simulink model "FLIGHT_hexacopter"  (R2024a)
settings: Solver=FixedStepDiscrete  StartTime=0.0  StopTime=inf  FixedStep=SampleTime_SAS  RelTol=1e-3  EnableMultiTasking=on
InitFcn:
  | Init_FLIGHT_Hexacopter
values from neighbouring files (symbols this model uses):
  d2r = pi/180    (= 0.0174532925199)    [Init_FLIGHT_Hexacopter.m]
  Kdpr = 0.004    [Init_FLIGHT_Hexacopter_fromNCMS.m]
  Kdrr = 0.004    [Init_FLIGHT_Hexacopter_fromNCMS.m]
  Kdvz = 0.0254    [Init_FLIGHT_Hexacopter_fromNCMS.m]
  Kdyr = 0.0298    [Init_FLIGHT_Hexacopter_fromNCMS.m]
  Kipr = 0.0    (= 0)    [Init_FLIGHT_Hexacopter_fromNCMS.m]
  Kirr = 0.0    (= 0)    [Init_FLIGHT_Hexacopter_fromNCMS.m]
  Kivz = 0.6304    [Init_FLIGHT_Hexacopter_fromNCMS.m]
  Kiyr = 0.0    (= 0)    [Init_FLIGHT_Hexacopter_fromNCMS.m]
  Kpp = 3.3894    [Init_FLIGHT_Hexacopter_fromNCMS.m]
  Kppr = 0.1    [Init_FLIGHT_Hexacopter_fromNCMS.m]
  Kpr = 3.3894    [Init_FLIGHT_Hexacopter_fromNCMS.m]
  Kprr = 0.1    [Init_FLIGHT_Hexacopter_fromNCMS.m]
  Kpvz = 0.3191    [Init_FLIGHT_Hexacopter_fromNCMS.m]
  Kpyr = 0.3744    [Init_FLIGHT_Hexacopter_fromNCMS.m]
  MAX_CONTROL_ANGLE_PITCH = 30*pi/180    (= 0.523598775598)    [Init_FLIGHT_Hexacopter.m]    (also in Init_FLIGHT_Hexacopter_fromNCMS.m = 0.349065850399)
  MAX_CONTROL_ANGLE_RATE_PITCH = 360*pi/180    (= 6.28318530718)    [Init_FLIGHT_Hexacopter.m]    (also in Init_FLIGHT_Hexacopter_fromNCMS.m)
  MAX_CONTROL_ANGLE_RATE_ROLL = 360*pi/180    (= 6.28318530718)    [Init_FLIGHT_Hexacopter.m]    (also in Init_FLIGHT_Hexacopter_fromNCMS.m)
  MAX_CONTROL_ANGLE_RATE_Y = 120*pi/180    (= 2.09439510239)    [Init_FLIGHT_Hexacopter.m]    (also in Init_FLIGHT_Hexacopter_fromNCMS.m)
  MAX_CONTROL_ANGLE_ROLL = 30*pi/180    (= 0.523598775598)    [Init_FLIGHT_Hexacopter.m]    (also in Init_FLIGHT_Hexacopter_fromNCMS.m = 0.349065850399)
  MAX_CONTROL_VELOCITY_XY = 1.5    [Init_FLIGHT_Hexacopter.m]    (also in Init_FLIGHT_Hexacopter_fromNCMS.m)
  MAX_CONTROL_VELOCITY_Z = 1    [Init_FLIGHT_Hexacopter.m]    (also in Init_FLIGHT_Hexacopter_fromNCMS.m)
  Npr = 50    [Init_FLIGHT_Hexacopter_fromNCMS.m]
  Nrr = 50    [Init_FLIGHT_Hexacopter_fromNCMS.m]
  Nvz = Npr    (= 50)    [Init_FLIGHT_Hexacopter_fromNCMS.m]
  Nyr = 50    [Init_FLIGHT_Hexacopter_fromNCMS.m]
  SampleTime = 1/200    (= 0.005)    [Init_FLIGHT_Hexacopter.m]    (also in Init_FLIGHT_Hexacopter_fromNCMS.m = 0.01)
  SampleTime_SAS = 1/1000    (= 0.001)    [Init_FLIGHT_Hexacopter.m]
undefined symbols (not defined in the file or in its folder): arguments, event_sequence, id, log_levels, MPC_Z_D, MPC_Z_I, MPC_Z_P, noutputs, output, pitch, pitch_body, q_d, roll, roll_body, thrust_body, timestamp, vx, vy, vz, x, y, yaw, yaw_sp_move_rate, z
libraries: px4lib x35, px4uORBlib x12, px4Utilslib x11, slpidlib x10, simulink x3, simulink_extras x2, px4Sensorslib x2, sharedtransform x1
(part 1 of 3)
settings Model: SimulationMode=external  ExtModeTrigDuration=10  Creator=user  LastModifiedBy=sslee
settings SolverCC: AlgebraicLoopSolver=TrustRegion  PositivePriorityOrder=on  MaxZcPerStep=1
settings OptimizationCC: DefaultUnderspecifiedDataType=single  EnhancedBackFolding=on  PassReuseOutputArgsAs=Individual arguments  ZeroExternalMemoryAtStartup=off  ZeroInternalMemoryAtStartup=off  MaxStackSize=64  OptimizeBlockOrder=speed  DifferentSizesBufferReuse=on  OptimizationCustomize=off  EfficientTunableParamExpr=on
settings DebuggingCC: ParameterTunabilityLossMsg=error  UnconnectedInputMsg=warning  UnconnectedOutputMsg=warning  UnconnectedLineMsg=warning
settings HardwareCC: ProdBitPerPointer=32  ProdBitPerSizeT=32  ProdBitPerPtrDiffT=32  ProdLargestAtomicInteger=Long  ProdLargestAtomicFloat=Double  ProdWordSize=32  ProdLongLongMode=on  ProdHWDeviceType=ARM Compatible->ARM Cortex
settings ModelReferenceCC: EnableRefExpFcnMdlSchedulingChecks=on
settings SFSimCC: MATLABDynamicMemAlloc=off  SimTargetLang=C++
settings RTWCC: Description=Embedded Coder  SystemTargetFile=ert.tlc  HardwareBoard=PX4 Pixhawk 6x  TLCOptions="-aInlineSetEventsForThisBaseRateFcn=TLC_FALSE -aSuppressMultiTaskScheduler=TLC_FALSE  -aRateBasedStepFcn=0"  TemplateMakefile=ert_default_tmf  GenerateReport=on  Toolchain=GNU Tools for PX4 Autopilots  TargetLang=C++  GPUComputeCapability=3.5  DLArmComputeVersion=19.05
settings CodeAppCC: ForceParamTrailComments=on  IgnoreCustomStorageClasses=off  OperatorAnnotations=on  SimulinkDataObjDesc=on  SFDataObjDesc=on  MATLABFcnDesc=on  InsertBlockDesc=on
settings ERTTargetCC: SupportVariableSizeSignals=on  ExtModeTransport=3  ExtModeStaticAlloc=on  ExtModeStaticAllocSize=1024  ExtModeMexFile=ext_xcp  ExtModeIntrfLevel=Level2 - Open

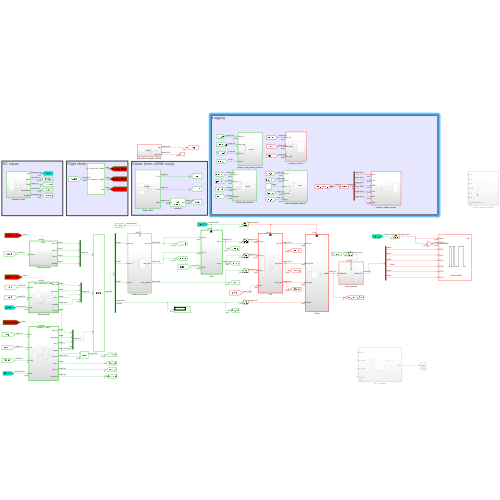
[thumbnail: Simulink's stored preview of the top-level diagram]
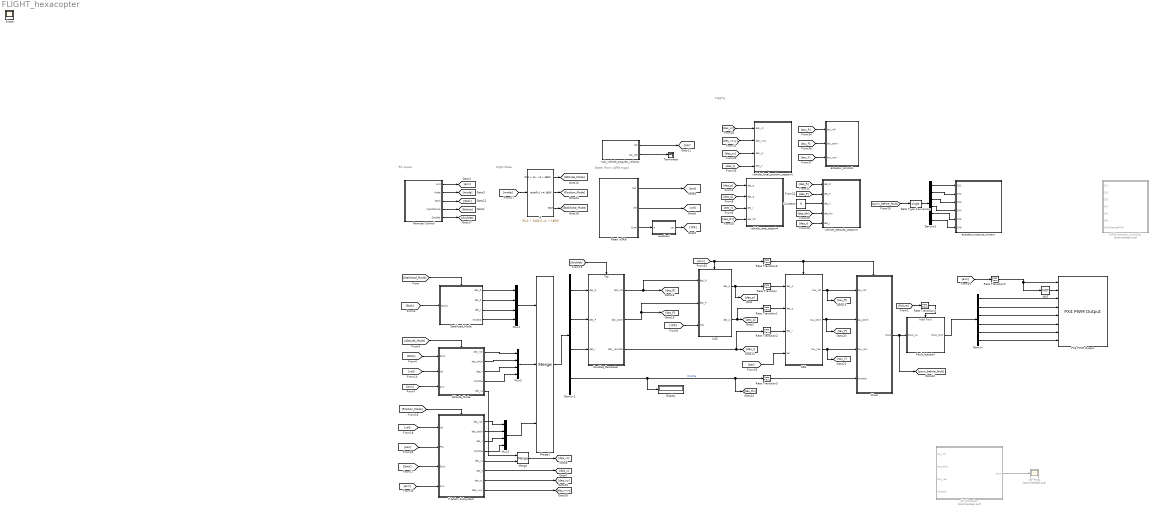
== system FLIGHT_hexacopter ==
  note: States (from uORB msgs)
  note: Logging
  note: Flight Mode
  note: RC inputs
  Altitude_Mode : Subsystem
  CAS : Subsystem
  Constant : Constant  Value=0  OutDataTypeStr=single  SampleTime=SampleTime
  Data Type Conversion : DataTypeConversion  OutDataTypeStr=single  SaturateOnIntegerOverflow=off  RndMeth=Floor
  Demux : Demux  Outputs=6
  Demux1 : Demux
  Demux3 : Demux  Outputs=6
  Display : Display
  Doublet_Generator : Subsystem
      settings: PortSchema="{\"entries\":[{\"content\":{\"sides\":[{\"content\":{\"connectorIds\":[\"In1\",\"In2\",\"In3\"]},\"type\":\"ConnectorPlacement.EquallySpacedRectSide\",\"uuid\":\"ec38b5d1-b3a9-4497-90eb-b31f6af6263d\"},{\"content\":{\"connectorIds\":[\"Out1\",\"Out2\",\"Out3\"],\"side\":\"RIGHT\"},\"type\":\"ConnectorPlacement.EquallySpacedRectSide\",\"uuid\":\"b680dd4c-5362-4b07-9f32-4954453bae35\"},{\"content\":{\"connectorIds\":[\"In4\"],\"side\":\"TOP\"},\"type\":\"ConnectorPlacement.EquallySpacedRectSide\",\"uuid\":\"c853e1a7-4b20-4202-99cf-4bec5916d7ea\"}]},\"type\":\"ConnectorPlacement.EquallySpacedConnector\",\"uuid\":\"c3796ba1-a87a-49a7-b842-2bb0a159edd5\"}],\"packageUris\":[\"http://schema.mathworks.com/mf0/Connector/R2020b\"],\"version\":\"1.0\"}"
  Fault_Injection : Subsystem
      settings: PortSchema="{\"entries\":[{\"content\":{\"sides\":[{\"content\":{\"connectorIds\":[\"In1\"]},\"type\":\"ConnectorPlacement.EquallySpacedRectSide\",\"uuid\":\"fab26c65-8d77-46b7-b375-2033d08e8306\"},{\"content\":{\"connectorIds\":[\"Out1\"],\"side\":\"RIGHT\"},\"type\":\"ConnectorPlacement.EquallySpacedRectSide\",\"uuid\":\"bc3f50bd-e170-4b75-8089-4f92da68e83e\"},{\"content\":{\"connectorIds\":[\"In2\"],\"side\":\"TOP\"},\"type\":\"ConnectorPlacement.EquallySpacedRectSide\",\"uuid\":\"873ada90-6f93-48ab-a701-a52d28357753\"}]},\"type\":\"ConnectorPlacement.EquallySpacedConnector\",\"uuid\":\"201be8b3-bff4-4924-8e0c-28e5fee33d1c\"}],\"packageUris\":[\"http://schema.mathworks.com/mf0/Connector/R2020b\"],\"version\":\"1.0\"}"
  If : If  IfExpression=u1 > 1400 & u1 < 1800  ElseIfExpressions=u1 >= 1800
  If Action Subsystem : Subsystem  TreatAsAtomicUnit=on
  Merge : Merge
  Merge1 : Merge  Inputs=3
  Mixer : Subsystem
  Mux1 : Mux
  Mux2 : Mux
  Mux3 : Mux
  NOT : Logic  Operator=NOT  IconShape=distinctive  AllPortsSameDT=off  OutDataTypeStr=boolean
  PX4 PWM Output : px4lib/PX4 PWM Output  pwmDevice=Main  pwmChannel1_=on  pwmChannel2_=on  pwmChannel3_=on  pwmChannel4_=on  pwmChannel5_=on  pwmChannel6_=on  pwmChannel7_=off  pwmChannel8_=off
      settings: SourceProductName=UAV Toolbox Support Package for PX4 Autopilots
  QP PWM : Scope  Commented=on
  QP_Allocation : Subsystem  Commented=on
  Rate Transition{,1..6} (7 alike) : RateTransition  OutPortSampleTime=SampleTime_SAS
  Read uORB : Subsystem
  Remote Control : Subsystem
  SAS : Subsystem
  Stabilized_Mode : Subsystem  TreatAsAtomicUnit=on
  Terminator : Terminator
  actuator_controls : Subsystem
  actuator_outputs_motors : Subsystem
  quat2eul : MATLAB Function  TreatAsAtomicUnit=on
  sub_vehicle_angular_velocity : Subsystem
  uORB_actuator_outputs1 : Subsystem  Commented=on
  vehicle_attitude_setpoint : Subsystem
  vehicle_local_position_setpoint : Subsystem
  vehicle_rate_setpoint : Subsystem
  Scope : Scope
  wires:
  Remote Control/4(InjectFailure) -> [failure]
  Stabilized_Mode/4(throttle) -> Mux1/4
  quat2eul/1(ypr) -> [YPR]
  [YPR] -> CAS/3(YPR)
  [mode] -> If/1
  sub_vehicle_angular_velocity/1(pqr) -> [pqr]
  [pqr] -> SAS/4(pqr)
  Read uORB/2(Vel) -> [vel]
  Mux1/1 -> Merge1/1
  Stabilized_Mode/2(des_P) -> Mux1/2
  Altitude_Mode/1(des_roll) -> Mux2/1
  Stabilized_Mode/1(des_R) -> Mux1/1
  Remote Control/2(Mode) -> [mode]
  Read uORB/3(Quat) -> quat2eul/1(q)
  Stabilized_Mode/3(des_r) -> Mux1/3
  Mux2/1 -> Merge1/2
  Altitude_Mode/3(des_r) -> Mux2/3
  Altitude_Mode/2(des_pitch) -> Mux2/2
  Demux1/4 -> Display/1, Rate Transition3/1, [des_thr]  "throttle"
  [Stick] -> Stabilized_Mode/1(Sticks)
  SAS/2(tau_pitch) -> [tau_P], Mixer/2(tau_pitch)
  SAS/1(tau_roll) -> [tau_R], Mixer/1(tau_roll)
  Remote Control/1(Arm) -> [arm]
  [Stick] -> Altitude_Mode/1(Stick)
  [Stabilized_Mode] -> Stabilized_Mode/Action
  [vel] -> Altitude_Mode/2(vel)
  SAS/3(tau_yaw) -> [tau_Y], Mixer/3(tau_yaw)
  If/1 -> [Altitude_Mode]
  CAS/1(des_p) -> [des_p], Rate Transition/1
  Merge1/1 -> Demux1/1
  If/3 -> [Stabilized_Mode]
  CAS/2(des_q) -> [des_q], Rate Transition1/1
  Fault_Injection/1(PWM_OUT) -> Demux/1
  Read uORB/1(Pos) -> [pos]
  Remote Control/3(Stick) -> [Stick]
  [Altitude_Mode] -> Altitude_Mode/Action
  [des_p] -> vehicle_rate_setpoint/1(des_p)
  [des_q] -> vehicle_rate_setpoint/2(des_q)
  [des_r] -> vehicle_rate_setpoint/3(des_r)
  [des_thr] -> vehicle_rate_setpoint/4(des_thr)
  Altitude_Mode/4(throttle) -> Mux2/4
  QP_Allocation/1(pwm) -> QP PWM/1
  Mixer/1(PWM) -> [pwm_before_fault], Fault_Injection/1(PWM_IN)
  Remote Control/5(Doublet) -> [doublet]
  [des_P] -> vehicle_attitude_setpoint/2(des_P)
  [des_R] -> vehicle_attitude_setpoint/1(des_R)
  [des_thr] -> vehicle_attitude_setpoint/4(des_thr)
  [des_r] -> vehicle_attitude_setpoint/5(des_r)
  [arm] -> Rate Transition5/1
  Demux/1 -> PX4 PWM Output/3
  Demux/2 -> PX4 PWM Output/4
  Demux/3 -> PX4 PWM Output/5
  Demux/4 -> PX4 PWM Output/6
  Demux/5 -> PX4 PWM Output/7
  Demux/6 -> PX4 PWM Output/8
  NOT/1 -> PX4 PWM Output/2
  Constant/1 -> vehicle_attitude_setpoint/3(des_Y)
  [pwm_before_fault] -> Data Type Conversion/1
  If/2 -> [Position_Mode]
  [Position_Mode] -> If Action Subsystem/Action
  [vel] -> If Action Subsystem/1(vel)
  If Action Subsystem/1(des_roll) -> Mux3/1
  If Action Subsystem/2(des_pitch) -> Mux3/2
  If Action Subsystem/3(des_r) -> Mux3/3
  If Action Subsystem/4(throttle) -> Mux3/4
  Mux3/1 -> Merge1/3
  Merge/1 -> [des_vz]
  Altitude_Mode/5(des_vz) -> Merge/1
  [des_vz] -> vehicle_local_position_setpoint/1(des_vz)
  [Stick] -> If Action Subsystem/3(Stick)
  [pos] -> If Action Subsystem/2(Pos)
  If Action Subsystem/5(des_vz) -> Merge/2
  If Action Subsystem/6(des_z) -> [des_z]
  If Action Subsystem/7(des_xy) -> [des_xy]
  If Action Subsystem/8(des_vxvy) -> [des_vxvy]
  [des_vxvy] -> vehicle_local_position_setpoint/2(des_vxvy)
  [des_xy] -> vehicle_local_position_setpoint/3(des_xy)
  [des_z] -> vehicle_local_position_setpoint/4(des_z)
  Data Type Conversion/1 -> Demux3/1
  [arm] -> Rate Transition6/1, CAS/Enable
  [arm] -> If Action Subsystem/4(arm)
  [arm] -> Altitude_Mode/3(arm)
  Demux3/1 -> actuator_outputs_motors/1(Ch1)
  Demux3/2 -> actuator_outputs_motors/2(Ch2)
  Demux3/3 -> actuator_outputs_motors/3(Ch3)
  Demux3/4 -> actuator_outputs_motors/4(Ch4)
  Demux3/5 -> actuator_outputs_motors/5(Ch5)
  Demux3/6 -> actuator_outputs_motors/6(Ch6)
  [tau_R] -> actuator_controls/1(tau_roll)
  [tau_P] -> actuator_controls/2(tau_pitch)
  [tau_Y] -> actuator_controls/3(tau_yaw)
  Demux1/1 -> Doublet_Generator/1(des_R)
  Demux1/2 -> Doublet_Generator/2(des_P)
  Demux1/3 -> Doublet_Generator/3(des_r)
  Doublet_Generator/1(des_roll) -> CAS/1(des_R), [des_R]
  Doublet_Generator/2(des_pitch) -> [des_P], CAS/2(des_P)
  Doublet_Generator/3(des_yawrate) -> [des_r], Rate Transition2/1
  [doublet] -> Doublet_Generator/4(flag)
  Rate Transition/1 -> SAS/1(des_p)
  Rate Transition1/1 -> SAS/2(des_q)
  Rate Transition2/1 -> SAS/3(des_r)
  Rate Transition3/1 -> Mixer/4(throttle)
  [failure] -> Rate Transition4/1
  Rate Transition4/1 -> Fault_Injection/2(Inject Fault)
  Rate Transition5/1 -> NOT/1, PX4 PWM Output/1
  Rate Transition6/1 -> SAS/Enable, Mixer/Enable
  sub_vehicle_angular_velocity/2(pqr_dot) -> Terminator/1

== system FLIGHT_hexacopter/Altitude_Mode ==
  Stick : Inport
  vel : Inport  Port=2
  arm : Inport  Port=3
  Action Port : ActionPort  ActionPortLabel=if(u1 > 1400 & u1 < 1800)
  Altitude_Mode_Stick2Command : Subsystem
  Demux2 : Demux  Outputs=3
  Terminator2 : Terminator
  Terminator3 : Terminator
  Vz Controller : Subsystem
  des_roll : Outport
  des_pitch : Outport  Port=2
  des_r : Outport  Port=3
  throttle : Outport  Port=4
  des_vz : Outport  Port=5
  wires:
  Stick/1 -> Altitude_Mode_Stick2Command/1(Stick)
  Vz Controller/1(throttle) -> throttle/1
  Demux2/3 -> Vz Controller/2(vz)
  vel/1 -> Demux2/1
  Altitude_Mode_Stick2Command/3(des_r) -> des_r/1
  Demux2/1 -> Terminator2/1
  Demux2/2 -> Terminator3/1
  Altitude_Mode_Stick2Command/2(des_pitch) -> des_pitch/1
  Altitude_Mode_Stick2Command/4(des_vz) -> des_vz/1, Vz Controller/1(des_vz)
  arm/1 -> Vz Controller/Enable
  Altitude_Mode_Stick2Command/1(des_roll) -> des_roll/1

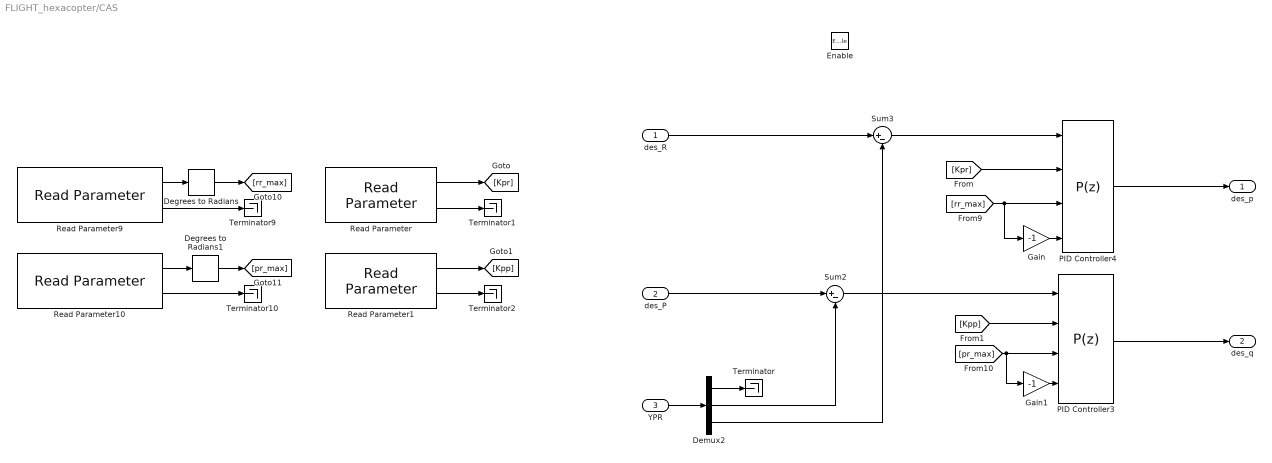
== system FLIGHT_hexacopter/CAS ==
  des_R : Inport
  des_P : Inport  Port=2
  YPR : Inport  Port=3
  Enable : EnablePort
  Degrees to Radians : simulink_extras/Transformations/Degrees to Radians
  Degrees to Radians1 : simulink_extras/Transformations/Degrees to Radians
  Demux2 : Demux  Outputs=3
  Gain : Gain  Gain=-1
  Gain1 : Gain  Gain=-1
  PID Controller3 : slpidlib/PID Controller  Controller=P  Form=Parallel  TimeDomain=Discrete-time  UseExternalTs=off  SampleTime=SampleTime  IntegratorMethod=Forward Euler  FilterMethod=Forward Euler  ControllerParametersSource=external  P=Kpp  I=1  UseKiTs=off  D=0  UseExternalDerivativeSource=off  N=100  UseFilter=on  TunerSelectOption=Transfer Function Based (PID Tuner App)  InitialConditionSource=internal  InitialConditionForIntegrator=0  InitialConditionForFilter=0  DifferentiatorICPrevScaledInput=0  ExternalReset=none  TrackingMode=off  Kt=1  LimitOutput=on  SatLimitsSource=external  UpperSaturationLimit=MAX_CONTROL_ANGLE_RATE_PITCH  LowerSaturationLimit=-MAX_CONTROL_ANGLE_RATE_PITCH  LinearizeAsGain=on  AntiWindupMode=none  Kb=1  LimitIntegrator=off  UpperIntegratorSaturationLimit=inf  LowerIntegratorSaturationLimit=-inf  POutMin=[]  POutMax=[]  IOutMin=[]  IOutMax=[]  DOutMin=[]  DOutMax=[]  NOutMin=[]  NOutMax=[]  SumOutMin=[]  SumOutMax=[]  SaturationOutMin=[]  SaturationOutMax=[]  PParamMin=[]  PParamMax=[]  IParamMin=[]  IParamMax=[]  DParamMin=[]  DParamMax=[]  NParamMin=[]  NParamMax=[]  KbParamMin=[]  KbParamMax=[]  KtParamMin=[]  KtParamMax=[]  KbOutMin=[]  KbOutMax=[]  KtOutMin=[]  KtOutMax=[]  IntegratorOutMin=[]  IntegratorOutMax=[]  FilterOutMin=[]  FilterOutMax=[]  SumI1OutMin=[]  SumI1OutMax=[]  SumI2OutMin=[]  SumI2OutMax=[]  SumI3OutMin=[]  SumI3OutMax=[]  SumI4OutMin=[]  SumI4OutMax=[]  SumDOutMin=[]  SumDOutMax=[]  DifferentiatorOutMin=[]  DifferentiatorOutMax=[]  FilterDiffOutCoefMin=[]  FilterDiffOutCoefMax=[]  ReciprocalOutMin=[]  ReciprocalOutMax=[]  SumDenOutMin=[]  SumDenOutMax=[]  SumNumOutMin=[]  SumNumOutMax=[]  DivideOutMin=[]  DivideOutMax=[]  UdiffTsProdOutMin=[]  UdiffTsProdOutMax=[]  NTsProdOutMin=[]  NTsProdOutMax=[]  UintegralTsProdOutMin=[]  UintegralTsProdOutMax=[]  UngainTsProdOutMin=[]  UngainTsProdOutMax=[]  ClampingZeroOutDataTypeStr=Inherit: Inherit via back propagation  ClampingZeroOutMin=[]  ClampingZeroOutMax=[]  FilterDenConstantOutDataTypeStr=Inherit: Inherit via back propagation  FilterDenConstantOutMin=[]  FilterDenConstantOutMax=[]  PCopyOutDataTypeStr=Inherit: Inherit via back propagation  PCopyOutMin=[]  PCopyOutMax=[]  NCopyOutDataTypeStr=Inherit: Inherit via back propagation  NCopyOutMin=[]  NCopyOutMax=[]  IntegratorContinuousStateAttributes=''  IntegratorStateMustResolveToSignalObject=off  IntegratorRTWStateStorageClass=Auto  FilterContinuousStateAttributes=''  FilterStateMustResolveToSignalObject=off  FilterRTWStateStorageClass=Auto  ParallelPVariant=ExternalParameters  IdealPVariant=Disabled  IVariant=Disabled  DVariant=Disabled  IntegratorVariant=Disabled  SatVariant=External  AWVariant=Disabled  PCopyVariant=Disabled  TRVariant=Disabled  FdbkBlocksVariant=Forward  IdealPFdbkVariant=Disabled  SatFdbkVariant=Disabled  DerivativeFilterVariant=Disabled  NVariant=Disabled  NCopyVariant=Disabled_SignalSpec  FilterICVariant=Disabled  IntegratorICVariant=Disabled  ExternalResetVariant=Disabled  TRSumVariant=Passthrough  SumFdbkVariant=Disabled  SumVariant=Passthrough_P  TsampFilterVariant=InternalTs  TsampNgainVariant=Passthrough  TsampIntegralVariant=Disabled_SignalSpec  ExternalSaturationOutDataTypeStr=Inherit: Same as second input  DerivativeSourceVariant=Disabled
  PID Controller4 : slpidlib/PID Controller  Controller=P  Form=Parallel  TimeDomain=Discrete-time  UseExternalTs=off  SampleTime=SampleTime  IntegratorMethod=Forward Euler  FilterMethod=Forward Euler  ControllerParametersSource=external  P=Kpr  I=1  UseKiTs=off  D=0  UseExternalDerivativeSource=off  N=100  UseFilter=on  TunerSelectOption=Transfer Function Based (PID Tuner App)  InitialConditionSource=internal  InitialConditionForIntegrator=0  InitialConditionForFilter=0  DifferentiatorICPrevScaledInput=0  ExternalReset=none  TrackingMode=off  Kt=1  LimitOutput=on  SatLimitsSource=external  UpperSaturationLimit=MAX_CONTROL_ANGLE_RATE_ROLL  LowerSaturationLimit=-MAX_CONTROL_ANGLE_RATE_ROLL  LinearizeAsGain=on  AntiWindupMode=none  Kb=1  LimitIntegrator=off  UpperIntegratorSaturationLimit=inf  LowerIntegratorSaturationLimit=-inf  POutMin=[]  POutMax=[]  IOutMin=[]  IOutMax=[]  DOutMin=[]  DOutMax=[]  NOutMin=[]  NOutMax=[]  SumOutMin=[]  SumOutMax=[]  SaturationOutMin=[]  SaturationOutMax=[]  PParamMin=[]  PParamMax=[]  IParamMin=[]  IParamMax=[]  DParamMin=[]  DParamMax=[]  NParamMin=[]  NParamMax=[]  KbParamMin=[]  KbParamMax=[]  KtParamMin=[]  KtParamMax=[]  KbOutMin=[]  KbOutMax=[]  KtOutMin=[]  KtOutMax=[]  IntegratorOutMin=[]  IntegratorOutMax=[]  FilterOutMin=[]  FilterOutMax=[]  SumI1OutMin=[]  SumI1OutMax=[]  SumI2OutMin=[]  SumI2OutMax=[]  SumI3OutMin=[]  SumI3OutMax=[]  SumI4OutMin=[]  SumI4OutMax=[]  SumDOutMin=[]  SumDOutMax=[]  DifferentiatorOutMin=[]  DifferentiatorOutMax=[]  FilterDiffOutCoefMin=[]  FilterDiffOutCoefMax=[]  ReciprocalOutMin=[]  ReciprocalOutMax=[]  SumDenOutMin=[]  SumDenOutMax=[]  SumNumOutMin=[]  SumNumOutMax=[]  DivideOutMin=[]  DivideOutMax=[]  UdiffTsProdOutMin=[]  UdiffTsProdOutMax=[]  NTsProdOutMin=[]  NTsProdOutMax=[]  UintegralTsProdOutMin=[]  UintegralTsProdOutMax=[]  UngainTsProdOutMin=[]  UngainTsProdOutMax=[]  ClampingZeroOutDataTypeStr=Inherit: Inherit via back propagation  ClampingZeroOutMin=[]  ClampingZeroOutMax=[]  FilterDenConstantOutDataTypeStr=Inherit: Inherit via back propagation  FilterDenConstantOutMin=[]  FilterDenConstantOutMax=[]  PCopyOutDataTypeStr=Inherit: Inherit via back propagation  PCopyOutMin=[]  PCopyOutMax=[]  NCopyOutDataTypeStr=Inherit: Inherit via back propagation  NCopyOutMin=[]  NCopyOutMax=[]  IntegratorContinuousStateAttributes=''  IntegratorStateMustResolveToSignalObject=off  IntegratorRTWStateStorageClass=Auto  FilterContinuousStateAttributes=''  FilterStateMustResolveToSignalObject=off  FilterRTWStateStorageClass=Auto  ParallelPVariant=ExternalParameters  IdealPVariant=Disabled  IVariant=Disabled  DVariant=Disabled  IntegratorVariant=Disabled  SatVariant=External  AWVariant=Disabled  PCopyVariant=Disabled  TRVariant=Disabled  FdbkBlocksVariant=Forward  IdealPFdbkVariant=Disabled  SatFdbkVariant=Disabled  DerivativeFilterVariant=Disabled  NVariant=Disabled  NCopyVariant=Disabled_SignalSpec  FilterICVariant=Disabled  IntegratorICVariant=Disabled  ExternalResetVariant=Disabled  TRSumVariant=Passthrough  SumFdbkVariant=Disabled  SumVariant=Passthrough_P  TsampFilterVariant=InternalTs  TsampNgainVariant=Passthrough  TsampIntegralVariant=Disabled_SignalSpec  ExternalSaturationOutDataTypeStr=Inherit: Same as second input  DerivativeSourceVariant=Disabled
  Read Parameter : px4lib/Read Parameter  ParameterName=MC_ROLL_P  DataType=FLOAT  SampleTime=SampleTime
      settings: SourceProductName=UAV Toolbox Support Package for PX4 Autopilots
  Read Parameter1 : px4lib/Read Parameter  ParameterName=MC_PITCH_P  DataType=FLOAT  SampleTime=SampleTime
      settings: SourceProductName=UAV Toolbox Support Package for PX4 Autopilots
  Read Parameter10 : px4lib/Read Parameter  ParameterName=MC_PITCHRATE_MAX  DataType=FLOAT  SampleTime=SampleTime
      settings: SourceProductName=UAV Toolbox Support Package for PX4 Autopilots
  Read Parameter9 : px4lib/Read Parameter  ParameterName=MC_ROLLRATE_MAX  DataType=FLOAT  SampleTime=SampleTime
      settings: SourceProductName=UAV Toolbox Support Package for PX4 Autopilots
  Sum2 : Sum  Inputs=|+-
  Sum3 : Sum  Inputs=|+-
  Terminator{,1..2,9..10} (5 alike) : Terminator
  des_p : Outport
  des_q : Outport  Port=2
  wires:
  Sum3/1 -> PID Controller4/1
  Sum2/1 -> PID Controller3/1
  Demux2/3 -> Sum3/2
  Demux2/2 -> Sum2/2
  YPR/1 -> Demux2/1
  Demux2/1 -> Terminator/1
  PID Controller4/1 -> des_p/1
  PID Controller3/1 -> des_q/1
  des_P/1 -> Sum2/1
  des_R/1 -> Sum3/1
  Read Parameter/2 -> Terminator1/1
  Read Parameter/1 -> [Kpr]
  Read Parameter1/1 -> [Kpp]
  Read Parameter1/2 -> Terminator2/1
  [Kpr] -> PID Controller4/2
  [Kpp] -> PID Controller3/2
  Degrees to Radians1/1 -> [pr_max]
  Read Parameter9/2 -> Terminator9/1
  Read Parameter10/1 -> Degrees to Radians1/1
  Read Parameter9/1 -> Degrees to Radians/1
  Read Parameter10/2 -> Terminator10/1
  Degrees to Radians/1 -> [rr_max]
  [rr_max] -> Gain/1, PID Controller4/3
  Gain/1 -> PID Controller4/4
  [pr_max] -> Gain1/1, PID Controller3/3
  Gain1/1 -> PID Controller3/4

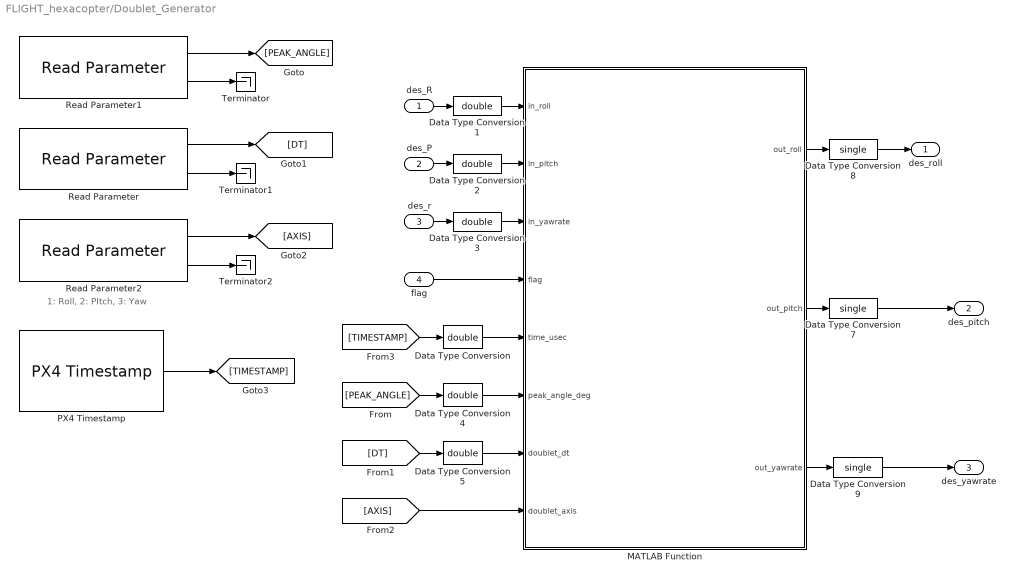
== system FLIGHT_hexacopter/Doublet_Generator ==
  note: 1: Roll, 2: PItch, 3: Yaw
  des_R : Inport
  des_P : Inport  Port=2
  des_r : Inport  Port=3
  flag : Inport  Port=4
  Data Type Conversion{,1..5} (6 alike) : DataTypeConversion  OutDataTypeStr=double  SaturateOnIntegerOverflow=off  RndMeth=Floor
  Data Type Conversion7 : DataTypeConversion  OutDataTypeStr=single  SaturateOnIntegerOverflow=off  RndMeth=Floor
  Data Type Conversion8 : DataTypeConversion  OutDataTypeStr=single  SaturateOnIntegerOverflow=off  RndMeth=Floor
  Data Type Conversion9 : DataTypeConversion  OutDataTypeStr=single  SaturateOnIntegerOverflow=off  RndMeth=Floor
  MATLAB Function : MATLAB Function  TreatAsAtomicUnit=on
  PX4 Timestamp : px4Utilslib/PX4 Timestamp  SampleTime=SampleTime
      settings: SourceProductName=PX4 Utility Blocks
  Read Parameter : px4lib/Read Parameter  ParameterName=DOUBLET_DT  DataType=FLOAT  SampleTime=SampleTime
      settings: SourceProductName=UAV Toolbox Support Package for PX4 Autopilots
  Read Parameter1 : px4lib/Read Parameter  ParameterName=DOUBLET_PEAK_ANG  DataType=FLOAT  SampleTime=SampleTime
      settings: SourceProductName=UAV Toolbox Support Package for PX4 Autopilots
  Read Parameter2 : px4lib/Read Parameter  ParameterName=DOUBLET_AXIS  DataType=INT32  SampleTime=SampleTime
      settings: SourceProductName=UAV Toolbox Support Package for PX4 Autopilots
  Terminator : Terminator
  Terminator1 : Terminator
  Terminator2 : Terminator
  des_roll : Outport
  des_pitch : Outport  Port=2
  des_yawrate : Outport  Port=3
  wires:
  Read Parameter1/2 -> Terminator/1
  Read Parameter/2 -> Terminator1/1
  Read Parameter2/2 -> Terminator2/1
  MATLAB Function/1(out_roll) -> Data Type Conversion8/1
  MATLAB Function/2(out_pitch) -> Data Type Conversion7/1
  MATLAB Function/3(out_yawrate) -> Data Type Conversion9/1
  des_R/1 -> Data Type Conversion1/1
  des_P/1 -> Data Type Conversion2/1
  des_r/1 -> Data Type Conversion3/1
  flag/1 -> MATLAB Function/4(flag)
  Read Parameter1/1 -> [PEAK_ANGLE]
  Read Parameter/1 -> [DT]
  Read Parameter2/1 -> [AXIS]
  [PEAK_ANGLE] -> Data Type Conversion4/1
  [DT] -> Data Type Conversion5/1
  PX4 Timestamp/1 -> [TIMESTAMP]
  [TIMESTAMP] -> Data Type Conversion/1
  Data Type Conversion/1 -> MATLAB Function/5(time_usec)
  Data Type Conversion1/1 -> MATLAB Function/1(in_roll)
  Data Type Conversion2/1 -> MATLAB Function/2(in_pitch)
  Data Type Conversion3/1 -> MATLAB Function/3(in_yawrate)
  Data Type Conversion4/1 -> MATLAB Function/6(peak_angle_deg)
  Data Type Conversion5/1 -> MATLAB Function/7(doublet_dt)
  Data Type Conversion8/1 -> des_roll/1
  Data Type Conversion7/1 -> des_pitch/1
  Data Type Conversion9/1 -> des_yawrate/1
  [AXIS] -> MATLAB Function/8(doublet_axis)

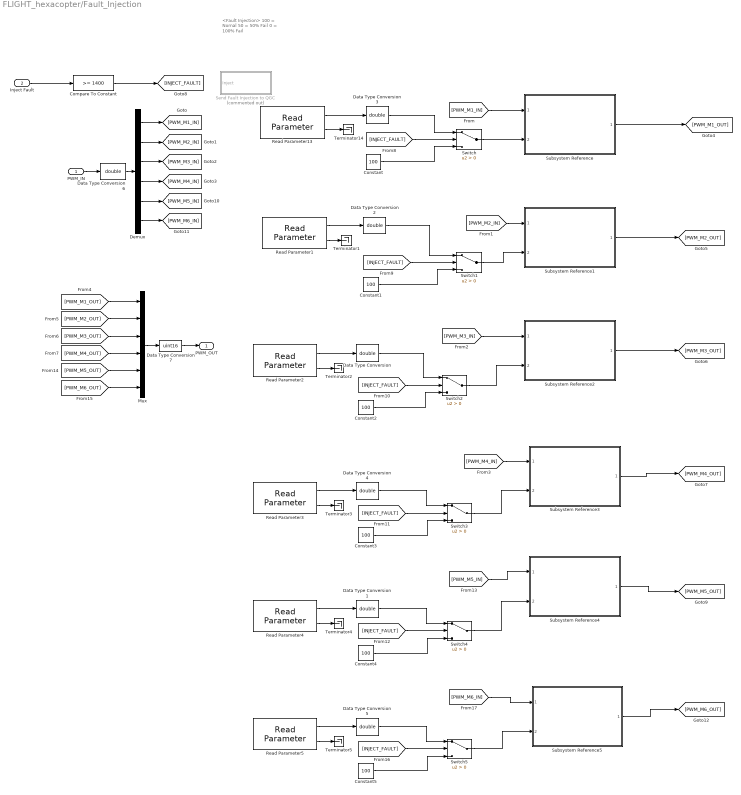
== system FLIGHT_hexacopter/Fault_Injection ==
  note: <Fault Injection>
      | 100 = Nornal
      | 50 = 50% Fail
      | 0 = 100% Fail
  PWM_IN : Inport
  Inject Fault : Inport  Port=2
  Compare To Constant : simulink/Logic and Bit Operations/Compare To Constant  relop=>=  const=1400  OutDataTypeStr=boolean
  Constant{,1..5} (6 alike) : Constant  Value=100
  Data Type Conversion{,1..6} (7 alike) : DataTypeConversion  OutDataTypeStr=double  SaturateOnIntegerOverflow=off  RndMeth=Floor
  Data Type Conversion7 : DataTypeConversion  OutDataTypeStr=uint16  SaturateOnIntegerOverflow=off  RndMeth=Floor
  Demux : Demux  Outputs=6
  Mux : Mux  Inputs=6
  Read Parameter1 : px4lib/Read Parameter  ParameterName=FDD_M2_STATUS  DataType=INT32  SampleTime=SampleTime_SAS
      settings: SourceProductName=UAV Toolbox Support Package for PX4 Autopilots
  Read Parameter13 : px4lib/Read Parameter  ParameterName=FDD_M1_STATUS  DataType=INT32  SampleTime=SampleTime_SAS
      settings: SourceProductName=UAV Toolbox Support Package for PX4 Autopilots
  Read Parameter2 : px4lib/Read Parameter  ParameterName=FDD_M3_STATUS  DataType=INT32  SampleTime=SampleTime_SAS
      settings: SourceProductName=UAV Toolbox Support Package for PX4 Autopilots
  Read Parameter3 : px4lib/Read Parameter  ParameterName=FDD_M4_STATUS  DataType=INT32  SampleTime=SampleTime_SAS
      settings: SourceProductName=UAV Toolbox Support Package for PX4 Autopilots
  Read Parameter4 : px4lib/Read Parameter  ParameterName=FDD_M5_STATUS  DataType=INT32  SampleTime=SampleTime_SAS
      settings: SourceProductName=UAV Toolbox Support Package for PX4 Autopilots
  Read Parameter5 : px4lib/Read Parameter  ParameterName=FDD_M6_STATUS  DataType=INT32  SampleTime=SampleTime_SAS
      settings: SourceProductName=UAV Toolbox Support Package for PX4 Autopilots
  Send Fault Injection to QGC : Subsystem  Commented=on  TreatAsAtomicUnit=on
  Subsystem Reference{,1..5} (6 alike) : Subsystem  ReferencedSubsystem=calculate_fault_injected_pwm
  Switch{,1..5} (6 alike) : Switch  Criteria=u2 > Threshold  SaturateOnIntegerOverflow=off  InputSameDT=off
  Terminator{1..5,14} (6 alike) : Terminator
  PWM_OUT : Outport
  wires:
  Read Parameter13/2 -> Terminator14/1
  Read Parameter1/2 -> Terminator1/1
  Read Parameter2/2 -> Terminator2/1
  Read Parameter2/1 -> Data Type Conversion/1
  Read Parameter3/2 -> Terminator3/1
  Read Parameter3/1 -> Data Type Conversion4/1
  Read Parameter13/1 -> Data Type Conversion3/1
  Read Parameter1/1 -> Data Type Conversion2/1
  Demux/1 -> [PWM_M1_IN]
  Demux/2 -> [PWM_M2_IN]
  Demux/3 -> [PWM_M3_IN]
  Demux/4 -> [PWM_M4_IN]
  Mux/1 -> Data Type Conversion7/1
  [PWM_M1_OUT] -> Mux/1
  [PWM_M2_OUT] -> Mux/2
  [PWM_M3_OUT] -> Mux/3
  [PWM_M4_OUT] -> Mux/4
  Inject Fault/1 -> Compare To Constant/1
  Compare To Constant/1 -> [INJECT_FAULT]
  Data Type Conversion3/1 -> Switch/1
  [INJECT_FAULT] -> Switch/2
  Constant/1 -> Switch/3
  Constant1/1 -> Switch1/3
  [INJECT_FAULT] -> Switch1/2
  Constant2/1 -> Switch2/3
  [INJECT_FAULT] -> Switch2/2
  Data Type Conversion/1 -> Switch2/1
  Constant3/1 -> Switch3/3
  [INJECT_FAULT] -> Switch3/2
  Data Type Conversion4/1 -> Switch3/1
  Read Parameter4/1 -> Data Type Conversion1/1
  Data Type Conversion1/1 -> Switch4/1
  Constant4/1 -> Switch4/3
  Read Parameter4/2 -> Terminator4/1
  [INJECT_FAULT] -> Switch4/2
  Demux/5 -> [PWM_M5_IN]
  Demux/6 -> [PWM_M6_IN]
  [PWM_M5_OUT] -> Mux/5
  [PWM_M6_OUT] -> Mux/6
  Data Type Conversion5/1 -> Switch5/1
  Read Parameter5/2 -> Terminator5/1
  [INJECT_FAULT] -> Switch5/2
  Read Parameter5/1 -> Data Type Conversion5/1
  Constant5/1 -> Switch5/3
  Data Type Conversion2/1 -> Switch1/1
  [PWM_M1_IN] -> Subsystem Reference/1
  Switch/1 -> Subsystem Reference/2
  [PWM_M2_IN] -> Subsystem Reference1/1
  Switch1/1 -> Subsystem Reference1/2
  [PWM_M3_IN] -> Subsystem Reference2/1
  Switch2/1 -> Subsystem Reference2/2
  Switch3/1 -> Subsystem Reference3/2
  [PWM_M4_IN] -> Subsystem Reference3/1
  [PWM_M5_IN] -> Subsystem Reference4/1
  Switch4/1 -> Subsystem Reference4/2
  [PWM_M6_IN] -> Subsystem Reference5/1
  Switch5/1 -> Subsystem Reference5/2
  Subsystem Reference/1 -> [PWM_M1_OUT]
  Subsystem Reference1/1 -> [PWM_M2_OUT]
  Subsystem Reference2/1 -> [PWM_M3_OUT]
  Subsystem Reference3/1 -> [PWM_M4_OUT]
  Subsystem Reference4/1 -> [PWM_M5_OUT]
  Subsystem Reference5/1 -> [PWM_M6_OUT]
  Data Type Conversion6/1 -> Demux/1
  PWM_IN/1 -> Data Type Conversion6/1
  Data Type Conversion7/1 -> PWM_OUT/1

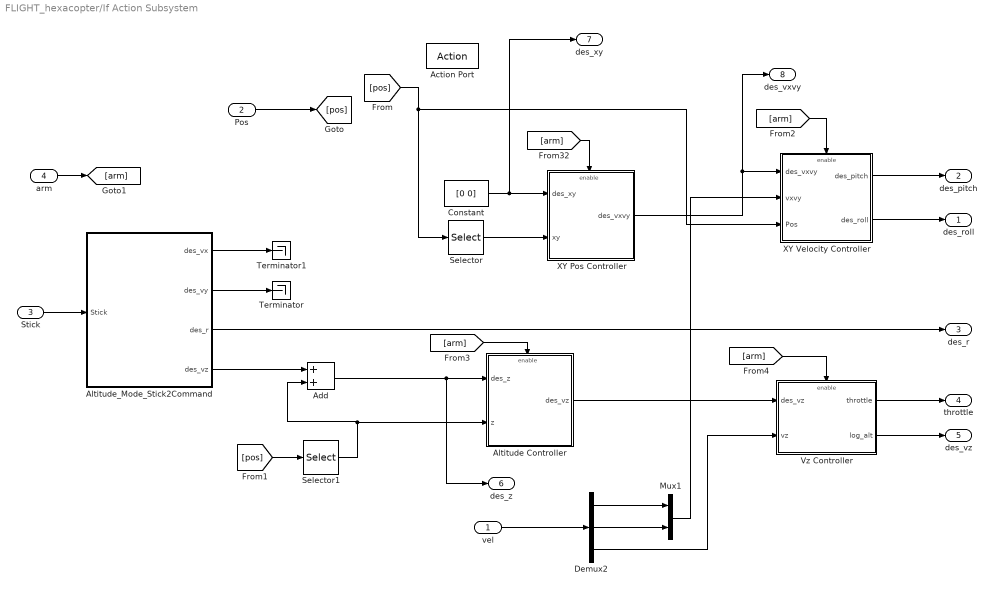
== system FLIGHT_hexacopter/If Action Subsystem ==
  vel : Inport
  Pos : Inport  Port=2
  Stick : Inport  Port=3
  arm : Inport  Port=4
  Action Port : ActionPort  ActionPortLabel=elseif(u1 >= 1800)
  Add : Sum
  Altitude Controller : Subsystem
  Altitude_Mode_Stick2Command : Subsystem
  Constant : Constant  Value=[0 0]  OutDataTypeStr=single
  Demux2 : Demux  Outputs=3
  Mux1 : Mux  Inputs=2
  Selector : Selector  InputPortWidth=4  IndexOptions=Index vector (dialog)  Indices=[1 2]  OutputSizes=1
  Selector1 : Selector  InputPortWidth=4  IndexOptions=Index vector (dialog)  Indices=3  OutputSizes=1
  Terminator : Terminator
  Terminator1 : Terminator
  Vz Controller : Subsystem
  XY Pos Controller : Subsystem
  XY Velocity Controller : Subsystem
  des_roll : Outport
  des_pitch : Outport  Port=2
  des_r : Outport  Port=3
  throttle : Outport  Port=4
  des_vz : Outport  Port=5
  des_z : Outport  Port=6
  des_xy : Outport  Port=7
  des_vxvy : Outport  Port=8
  wires:
  Demux2/2 -> Mux1/2
  Altitude_Mode_Stick2Command/3(des_r) -> des_r/1
  Vz Controller/2(log_alt) -> des_vz/1
  Vz Controller/1(throttle) -> throttle/1
  Demux2/3 -> Vz Controller/2(vz)
  vel/1 -> Demux2/1
  Demux2/1 -> Mux1/1
  Mux1/1 -> XY Velocity Controller/2(vxvy)
  XY Velocity Controller/1(des_pitch) -> des_pitch/1
  XY Velocity Controller/2(des_roll) -> des_roll/1
  Stick/1 -> Altitude_Mode_Stick2Command/1(Stick)
  Selector/1 -> XY Pos Controller/2(xy)
  XY Pos Controller/1(des_vxvy) -> des_vxvy/1, XY Velocity Controller/1(des_vxvy)
  Pos/1 -> [pos]
  [pos] -> XY Velocity Controller/3(Pos), Selector/1
  Altitude Controller/1(des_vz) -> Vz Controller/1(des_vz)
  Altitude_Mode_Stick2Command/4(des_vz) -> Add/1
  [pos] -> Selector1/1
  Selector1/1 -> Add/2, Altitude Controller/2(z)
  Add/1 -> des_z/1, Altitude Controller/1(des_z)
  Altitude_Mode_Stick2Command/2(des_vy) -> Terminator/1
  Altitude_Mode_Stick2Command/1(des_vx) -> Terminator1/1
  Constant/1 -> des_xy/1, XY Pos Controller/1(des_xy)
  [arm] -> XY Pos Controller/Enable
  [arm] -> XY Velocity Controller/Enable
  [arm] -> Altitude Controller/Enable
  [arm] -> Vz Controller/Enable
  arm/1 -> [arm]

== system FLIGHT_hexacopter/Mixer ==
  tau_roll : Inport
  tau_pitch : Inport  Port=2
  tau_yaw : Inport  Port=3
  throttle : Inport  Port=4
  Enable : EnablePort
  Mux : Mux  Inputs=6
  Output_Limits1 : Saturate  UpperLimit=2000  LowerLimit=1000  OutDataTypeStr=uint16
  pwm_out2 : MATLAB Function  SystemSampleTime=0.004
  PWM : Outport
  wires:
  tau_yaw/1 -> pwm_out2/3(Yaw)
  throttle/1 -> pwm_out2/4(Thrust)
  tau_roll/1 -> pwm_out2/1(Roll)
  pwm_out2/5(M5) -> Mux/5
  pwm_out2/6(M6) -> Mux/6
  tau_pitch/1 -> pwm_out2/2(Pitch)
  pwm_out2/4(M4) -> Mux/4
  pwm_out2/2(M2) -> Mux/2
  pwm_out2/3(M3) -> Mux/3
  pwm_out2/1(M1) -> Mux/1
  Output_Limits1/1 -> PWM/1
  Mux/1 -> Output_Limits1/1

== system FLIGHT_hexacopter/QP_Allocation ==
  tau_roll : Inport
  tau_pitch : Inport  Port=2
  tau_yaw : Inport  Port=3
  throttle : Inport  Port=4
  Add : Sum
  Constant : Constant  Value=[1; 1; 1; 1; 1; 1]
  Constant1 : Constant  Value=[1 1 1 1 1 1; 0.275 -0.275 0.1375 -0.1375 -0.1375 0.1375; 0 0 0.2382 -0.2382 0.2382 -0.2382; -0.1 0.1 -0.1 0.1 -0.1 0.1]
  Constant2 : Constant  Value=1000
  Data Type Conversion : DataTypeConversion  OutDataTypeStr=single  SaturateOnIntegerOverflow=off  RndMeth=Floor
  Delay : Delay  DelayLength=1
  Gain : Gain  Gain=1000
  Gain1 : Gain  Gain=10
  Gain2 : Gain  Gain=2
  Gain3 : Gain
  Gain4 : Gain
  MATLAB Function : MATLAB Function  TreatAsAtomicUnit=on
  pwm : Outport
  wires:
  MATLAB Function/2(thrust_setpoints) -> Delay/1
  Delay/1 -> MATLAB Function/6(u_prev)
  Constant1/1 -> MATLAB Function/5(A)
  Constant/1 -> MATLAB Function/7(failure_status)
  throttle/1 -> Gain1/1
  tau_roll/1 -> Gain2/1
  tau_pitch/1 -> Gain3/1
  tau_yaw/1 -> Gain4/1
  MATLAB Function/1(normalized_thrust_setpoint) -> Gain/1
  Gain/1 -> Add/1
  Constant2/1 -> Add/2
  Add/1 -> Data Type Conversion/1
  Data Type Conversion/1 -> pwm/1
  Gain1/1 -> MATLAB Function/1(f_total)
  Gain2/1 -> MATLAB Function/2(tau_phi)
  Gain3/1 -> MATLAB Function/3(tau_theta)
  Gain4/1 -> MATLAB Function/4(tau_psi)

== system FLIGHT_hexacopter/Read uORB ==
  Bus Selector : BusSelector  OutputSignals=x,y,z,heading  OutputAsBus=on
  Bus Selector1 : BusSelector  OutputSignals=vx,vy,vz  OutputAsBus=on
  Data Type Conversion : DataTypeConversion  OutDataTypeStr=single  SaturateOnIntegerOverflow=off  RndMeth=Floor
  Data Type Conversion9 : DataTypeConversion  OutDataTypeStr=single  SaturateOnIntegerOverflow=off  RndMeth=Floor
  PX4 uORB Read : px4uORBlib/PX4 uORB Read  uORBTopic=VehicleLocalPosition  selectInstance=vehicle_local_position  SampleTime=SampleTime  BlockingMode=off  BlockTimeout=1e-3
      settings: SourceProductName=PX4 uORB Read and Write Blocks
  Terminator : Terminator
  Terminator5 : Terminator
  Vehicle Attitude : px4Sensorslib/Vehicle Attitude  rollRate=off  pitchRate=off  yawRate=off  quaternion=on  uorbTimeStamp=off  BlockingMode=off  BlockTimeout=0.001  sampleTime=SampleTime
  Pos : Outport
  Vel : Outport  Port=2
  Quat : Outport  Port=3
  wires:
  Vehicle Attitude/1 -> Terminator5/1
  PX4 uORB Read/1 -> Terminator/1
  PX4 uORB Read/2 -> Bus Selector1/1, Bus Selector/1
  Vehicle Attitude/2 -> Quat/1
  Bus Selector1/1 -> Data Type Conversion9/1
  Bus Selector/1 -> Data Type Conversion/1
  Data Type Conversion/1 -> Pos/1
  Data Type Conversion9/1 -> Vel/1

== system FLIGHT_hexacopter/Remote Control ==
  Arm1 : Subsystem
  Compare To Constant : simulink/Logic and Bit Operations/Compare To Constant  relop=>=  const=1800  OutDataTypeStr=boolean
  Mux3 : Mux
  Radio Control Transmitter : px4Sensorslib/Radio Control Transmitter  channel1=on  channel2=on  channel3=on  channel4=on  channel5=on  channel6=on  channel7=on  channel8=on  channel_count=off  rssi=off  rc_input_source=off  timestamp_last_signal=off  time_stamp=off  sampleTime=SampleTime  BlockingMode=off  BlockTimeout=5
  Terminator1 : Terminator
  Arm : Outport
  Mode : Outport  Port=2
  Stick : Outport  Port=3
  InjectFailure : Outport  Port=4
  Doublet : Outport  Port=5
  wires:
  Mux3/1 -> Stick/1
  Radio Control Transmitter/1 -> Terminator1/1
  Radio Control Transmitter/7 -> Mode/1  "mode_signal"
  Radio Control Transmitter/5 -> Mux3/3  "des_Y"
  Radio Control Transmitter/9 -> InjectFailure/1
  Radio Control Transmitter/2 -> Mux3/1  "des_R"
  Radio Control Transmitter/3 -> Mux3/2  "des_P"
  Radio Control Transmitter/8 -> Compare To Constant/1
  Radio Control Transmitter/6 -> Arm1/1(Arm)  "arm_signal"
  Arm1/1(Arm_cmd) -> Arm/1
  Radio Control Transmitter/4 -> Mux3/4  "throttle, des_vz"
  Compare To Constant/1 -> Doublet/1
